simulink model "part_2_coulomb_friction"  (R2019a)
settings: Solver=VariableStepAuto  StartTime=0.0  StopTime=9  RelTol=1e-3
libraries: simulink x1
settings Model: Creator=Matthew Frantz  LastModifiedBy=Matthew Frantz
settings SolverCC: ZeroCrossAlgorithm=Adaptive
settings DebuggingCC: IgnoredZcDiagnostic=none

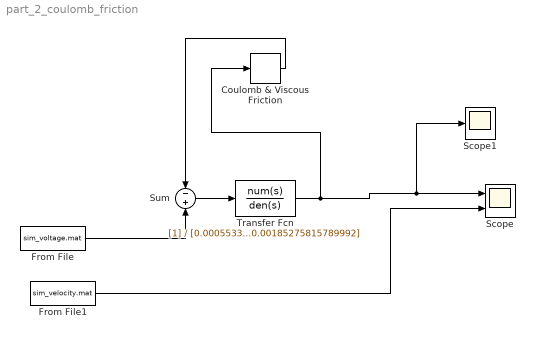
== system part_2_coulomb_friction ==
  Coulomb & Viscous Friction : simulink/Discontinuities/Coulomb & Viscous Friction  offset=0.138247141541477  gain=0
      settings: SourceProductName=Simulink
  From File : FromFile  FileName=sim_voltage.mat  SampleTime=0
  From File1 : FromFile  FileName=sim_velocity.mat  SampleTime=0
  Scope : Scope  NumInputPorts=2
  Scope1 : Scope
  Sum : Sum  Inputs=-+
  Transfer Fcn : TransferFcn  Denominator=[0.000553342193254858 0.00185275815789992]
  wires:
  Transfer Fcn/1 -> Coulomb & Viscous Friction/1, Scope1/1, Scope/1
  From File1/1 -> Scope/2
  Sum/1 -> Transfer Fcn/1
  From File/1 -> Sum/2
  Coulomb & Viscous Friction/1 -> Sum/1
